simulink model "mileston_7"  (R2020b)
settings: Solver=VariableStepAuto  StartTime=0.0  StopTime=10.0  RelTol=1e-3
libraries: simulink x1
settings Model: Creator=admin  LastModifiedBy=admin

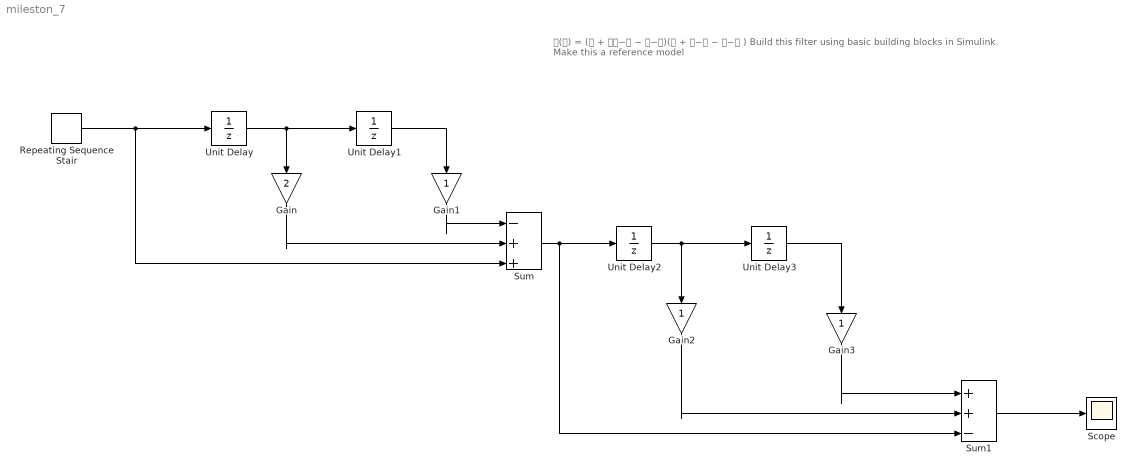
== system mileston_7 ==
  note: 𝐇(𝐳) = (𝟏 + 𝟐𝐳−𝟏 − 𝐳−𝟐)(𝟏 + 𝐳−𝟏 − 𝐳−𝟐 )
      | Build this filter using basic building blocks in Simulink. Make this a reference model
  Gain : Gain  Gain=2
  Gain1 : Gain
  Gain2 : Gain
  Gain3 : Gain
  Repeating Sequence Stair : simulink/Sources/Repeating Sequence Stair  OutValues=[3 1 4 2 1].'  tsamp=-1  OutMin=[]  OutMax=[]  OutDataTypeStr=double  OutputDataTypeScalingMode=double  OutDataType=fixdt(0,8)  ConRadixGroup=Best Precision: Vector-wise  OutScaling=2^-12
  Scope : Scope
  Sum : Sum  Inputs=|-++
  Sum1 : Sum  Inputs=|++-
  Unit Delay{,1..3} (4 alike) : UnitDelay  SampleTime=-1  HasFrameUpgradeWarning=on
  wires:
  Repeating Sequence Stair/1 -> Sum/3, Unit Delay/1
  Unit Delay/1 -> Gain/1, Unit Delay1/1
  Unit Delay1/1 -> Gain1/1
  Gain1/1 -> Sum/1
  Gain/1 -> Sum/2
  Sum/1 -> Unit Delay2/1, Sum1/3
  Unit Delay2/1 -> Unit Delay3/1, Gain2/1
  Unit Delay3/1 -> Gain3/1
  Gain3/1 -> Sum1/1
  Gain2/1 -> Sum1/2
  Sum1/1 -> Scope/1
